simulink model "model_transmitancja"  (R2023b)
settings: Solver=ode4  StartTime=0.0  StopTime=5000.0  FixedStep=0.1  RelTol=1e-3
settings Model: Creator=tototmek  LastModifiedBy=tototmek

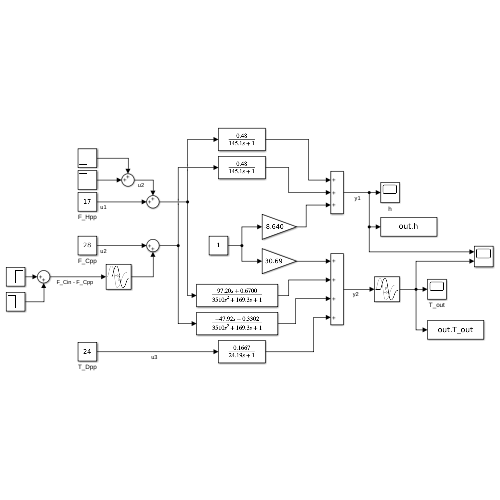
[thumbnail: Simulink's stored preview of the top-level diagram]
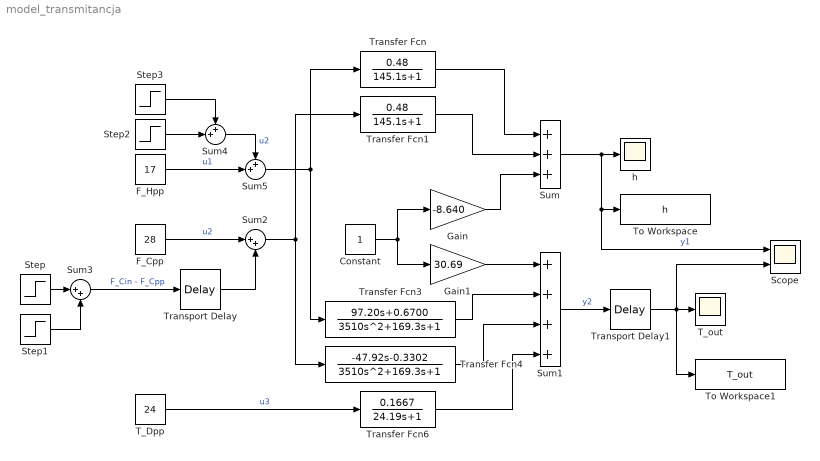
== system model_transmitancja ==
  Constant : Constant
  F_Cpp : Constant  Value=28
  F_Hpp : Constant  Value=17
  Gain : Gain  Gain=-8.640
  Gain1 : Gain  Gain=30.69
  Scope : Scope  NumInputPorts=2
  Step : Step  Time=2000  After=2.8  SampleTime=0
  Step1 : Step  Time=2500  After=-5.6  SampleTime=0
  Step2 : Step  Time=1500  After=-3.4  SampleTime=0
  Step3 : Step  Time=1000  After=1.7  SampleTime=0
  Sum : Sum  Inputs=+++
  Sum1 : Sum  Inputs=++++
  Sum2 : Sum  Inputs=|++
  Sum3 : Sum  Inputs=|++
  Sum4 : Sum  Inputs=++|
  Sum5 : Sum  Inputs=++|
  T_Dpp : Constant  Value=24
  T_out : Scope
  To Workspace : ToWorkspace  VariableName=h  SaveFormat=Timeseries  SampleTime=-1
  To Workspace1 : ToWorkspace  VariableName=T_out  SaveFormat=Timeseries  SampleTime=-1
  Transfer Fcn : TransferFcn  Numerator=[0.48]  Denominator=[145.1 1]
  Transfer Fcn1 : TransferFcn  Numerator=[0.48]  Denominator=[145.1 1]
  Transfer Fcn3 : TransferFcn  Numerator=[97.20 0.6700]  Denominator=[3510 169.3 1]
  Transfer Fcn4 : TransferFcn  Numerator=[-47.92 -0.3302]  Denominator=[3510 169.3 1]
  Transfer Fcn6 : TransferFcn  Numerator=[0.1667]  Denominator=[24.19 1]
  Transport Delay : TransportDelay  DelayTime=90
  Transport Delay1 : TransportDelay  DelayTime=40
  h : Scope
  wires:
  Gain/1 -> Sum/3
  Sum5/1 -> Transfer Fcn/1, Transfer Fcn3/1
  Sum2/1 -> Transfer Fcn1/1, Transfer Fcn4/1
  Transfer Fcn1/1 -> Sum/2
  Transfer Fcn/1 -> Sum/1
  Sum/1 -> Scope/1, To Workspace/1, h/1  "y1"
  Gain1/1 -> Sum1/1
  Constant/1 -> Gain/1, Gain1/1
  Transfer Fcn3/1 -> Sum1/2
  Transfer Fcn4/1 -> Sum1/3
  Sum1/1 -> Transport Delay1/1  "y2"
  F_Cpp/1 -> Sum2/1  "u2"
  Step1/1 -> Sum3/2
  Step3/1 -> Sum4/1
  Step/1 -> Sum3/1
  Sum3/1 -> Transport Delay/1  "F_Cin - F_Cpp"
  Transport Delay/1 -> Sum2/2
  Transport Delay1/1 -> To Workspace1/1, Scope/2, T_out/1
  F_Hpp/1 -> Sum5/2  "u1"
  Step2/1 -> Sum4/2
  Sum4/1 -> Sum5/1  "u2"
  T_Dpp/1 -> Transfer Fcn6/1  "u3"
  Transfer Fcn6/1 -> Sum1/4
